simulink model "MRG1x_17B_ERP_030_00_Star23_xx_M256xx_910_x64_RB_Test"  (Simulink 7.8)
settings: Solver=ode45  SolverMode=SingleTasking  StartTime=0.0  StopTime=10.0  RelTol=1e-3
PreLoadFcn:
  | MRG1x_17B_ERP_030_00_Star23_xx_M256xx_910_x64_InitFcn
undefined symbols (not defined in the file or in its folder): ECM
(part 1 of 2)
settings Model: Creator=Silver 3.4.1759  LastModifiedBy=vpadmaj
settings OptimizationCC: BlockReduction=off  BooleanDataType=off
settings DebuggingCC: SaveWithParameterizedLinksMsg=none  SignalResolutionControl=TryResolveAllWithWarning  SolverPrmCheckMsg=none  StrictBusMsg=Warning
settings HardwareCC: TargetUnknown=on

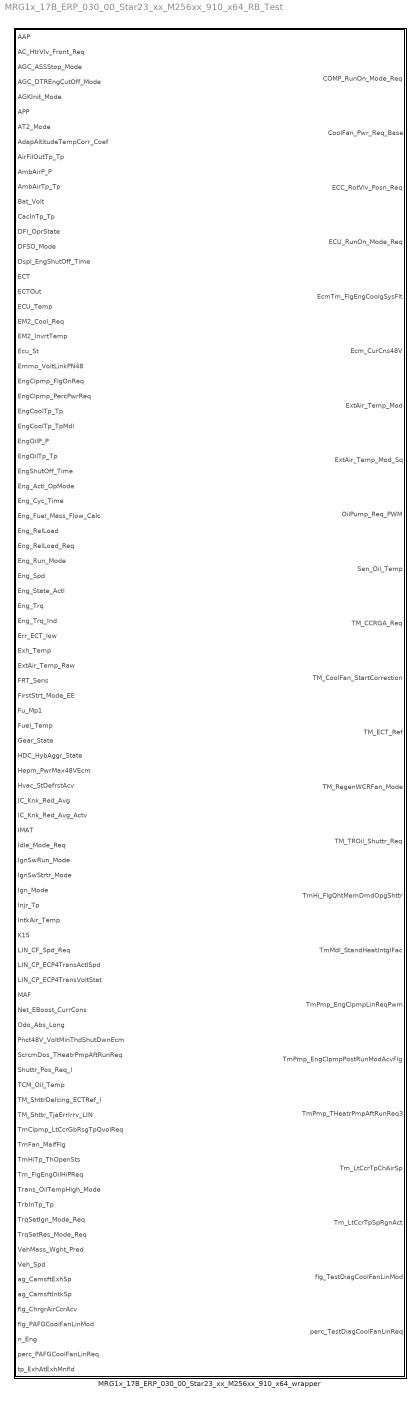
== system MRG1x_17B_ERP_030_00_Star23_xx_M256xx_910_x64_RB_Test ==
  MRG1x_17B_ERP_030_00_Star23_xx_M256xx_910_x64_wrapper : Subsystem
      mask Display:
      | patch(.5 + 0.03*8*cos(0:pi/50:2*pi),   .5 + 0.0753 *8*sin(0:pi/50:2*pi), [0 0 1])
      | patch(.5 + 0.03*[6.5, 8, 0, -1.5],     .5 + 0.0753 *[-8,-6.5, 1.5, 0], [.8, .8, .8])
      | patch(.5 + 0.03*5.5*cos(0:pi/50:2*pi), .5 + 0.0753 *5.5*sin(0:pi/50:2*pi), [.8, .8, .8])
      | patch(.5 + 0.03*3.5*cos(0:pi/50:2*pi), .5 + 0.0753 *3.5*sin(0:pi/50:2*pi), [0 0 1])
